simulink model "CommsInCustom"  (R2026a)
settings: Solver=VariableStepAuto
libraries: simulink x3, etargetslib x1
settings Model: DataDictionary=QuadData.sldd  Creator=The MathWorks, Inc.  LastModifiedBy=The MathWorks, Inc.

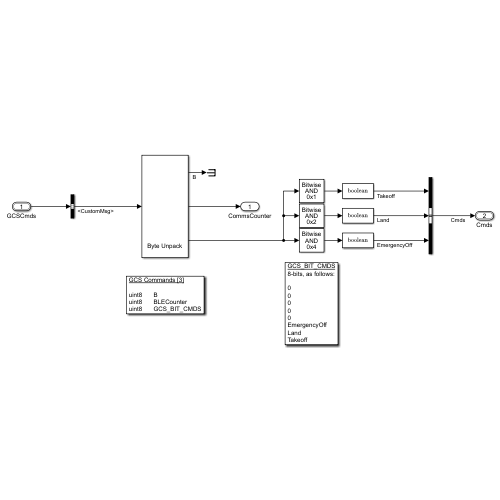
[thumbnail: Simulink's stored preview of the top-level diagram]
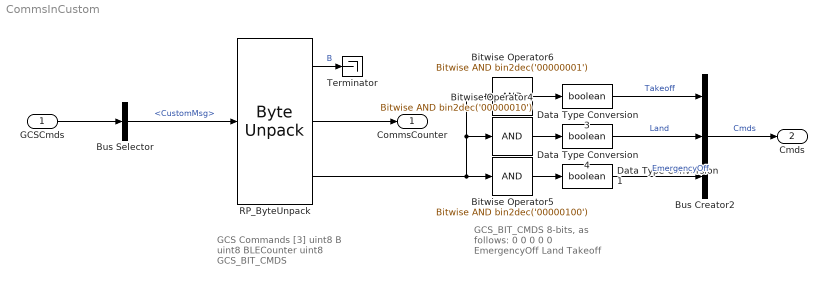
== system CommsInCustom ==
  note: GCS_BIT_CMDS
      | 8-bits, as follows:
      |
      | 0
      | 0
      | 0
      | 0
      | 0
      | EmergencyOff
      | Land
      | Takeoff
  note: GCS Commands [3]
      |
      | uint8 B
      | uint8 BLECounter
      | uint8 GCS_BIT_CMDS
  GCSCmds : Inport  OutDataTypeStr=Bus: GCSCmds  BusOutputAsStruct=on
  Bitwise Operator4 : simulink/Logic and Bit Operations/Bitwise Operator  logicop=AND  UseBitMask=on  BitMask=bin2dec('00000010')  BitMaskRealWorld=Stored Integer
  Bitwise Operator5 : simulink/Logic and Bit Operations/Bitwise Operator  logicop=AND  UseBitMask=on  BitMask=bin2dec('00000100')  BitMaskRealWorld=Stored Integer
  Bitwise Operator6 : simulink/Logic and Bit Operations/Bitwise Operator  logicop=AND  UseBitMask=on  BitMask=bin2dec('00000001')  BitMaskRealWorld=Stored Integer
  Bus Creator2 : BusCreator  Inputs=3  OutDataTypeStr=Bus: Cmds  NonVirtualBus=on
  Bus Selector : BusSelector  OutputSignals=CustomMsg
  Data Type Conversion1 : DataTypeConversion  OutDataTypeStr=boolean  SaturateOnIntegerOverflow=off  RndMeth=Floor
  Data Type Conversion3 : DataTypeConversion  OutDataTypeStr=boolean  SaturateOnIntegerOverflow=off  RndMeth=Floor
  Data Type Conversion4 : DataTypeConversion  OutDataTypeStr=boolean  SaturateOnIntegerOverflow=off  RndMeth=Floor
  RP_ByteUnpack : etargetslib/Byte Unpack  dimensions={[1] [1] [1]}  datatypes={'uint8' 'uint8' 'uint8'}  byteAlign=1
  Terminator : Terminator
  CommsCounter : Outport  OutDataTypeStr=uint8  PortDimensions=1  VectorParamsAs1DForOutWhenUnconnected=off
  Cmds : Outport  Port=2  OutDataTypeStr=Bus: Cmds  VectorParamsAs1DForOutWhenUnconnected=off
  wires:
  Data Type Conversion4/1 -> Bus Creator2/2  "Land"
  Data Type Conversion1/1 -> Bus Creator2/3  "EmergencyOff"
  RP_ByteUnpack/2 -> CommsCounter/1
  Data Type Conversion3/1 -> Bus Creator2/1  "Takeoff"
  Bus Creator2/1 -> Cmds/1  "Cmds"
  RP_ByteUnpack/3 -> Bitwise Operator6/1, Bitwise Operator4/1, Bitwise Operator5/1
  Bitwise Operator6/1 -> Data Type Conversion3/1
  RP_ByteUnpack/1 -> Terminator/1  "B"
  Bitwise Operator4/1 -> Data Type Conversion4/1
  Bitwise Operator5/1 -> Data Type Conversion1/1
  GCSCmds/1 -> Bus Selector/1
  Bus Selector/1 -> RP_ByteUnpack/1  "<CustomMsg>"
